simulink model "G_actuatordynamics"  (R2017a)
settings: Solver=FixedStepAuto  StartTime=0.0  StopTime=10  FixedStep=sim_time  RelTol=1e-3  EnableMultiTasking=on
values from neighbouring files (symbols this model uses):
  B = [1 0.5 -0.5 -1 0 0.5 ; 0 0 0 0 2 0 ; -0.05 -0.02 0.02 0.05 0 2 ; -1 -1 -1 -1 -2 0]    [A_runSimulation.m]    (also in C_runSimulation.m; D_runSimulation.m; E_runSimulation.m; F_runSimulation.m)
  gain_four = rand()*2    [A_runSimulation.m]    (also in C_runSimulation.m = 0; D_runSimulation.m; E_runSimulation.m = 0; F_runSimulation.m = 0)
  gain_one = rand()*2    [A_runSimulation.m]    (also in C_runSimulation.m = 0; D_runSimulation.m; E_runSimulation.m = 0; F_runSimulation.m = 0)
  gain_three = rand()*2    [A_runSimulation.m]    (also in C_runSimulation.m = 0; D_runSimulation.m; E_runSimulation.m = 0; F_runSimulation.m = 0)
  gain_two = rand()*2    [A_runSimulation.m]    (also in C_runSimulation.m = 0; D_runSimulation.m; E_runSimulation.m = 0; F_runSimulation.m = 0)
  seed_four = k + 30    [A_runSimulation.m]    (also in C_runSimulation.m; D_runSimulation.m; E_runSimulation.m; F_runSimulation.m)
  seed_one = k    [A_runSimulation.m]    (also in C_runSimulation.m; D_runSimulation.m; E_runSimulation.m; F_runSimulation.m)
  seed_three = k + 20    [A_runSimulation.m]    (also in C_runSimulation.m; D_runSimulation.m; E_runSimulation.m; F_runSimulation.m)
  seed_two = k + 10    [A_runSimulation.m]    (also in C_runSimulation.m; D_runSimulation.m; E_runSimulation.m; F_runSimulation.m)
  signal_gain = j    [A_runSimulation.m]    (also in C_runSimulation.m; D_runSimulation.m; E_runSimulation.m = 0.3; F_runSimulation.m)
  sim_time = 1    [E_runSimulation.m]    (also in F_runSimulation.m = 0.1; F_runSimulation2.m = 0.1; G_runSimulation.m = 0.001)
  u_lim = [[-0.5 -0.5 -0.5 -0.5 -0.5 -0.5]' [0.5 0.5 0.5 0.5 0.5 0.5]']    [A_runSimulation.m]    (also in C_runSimulation.m; D_runSimulation.m; E_runSimulation.m; F_runSimulation.m)
  udot_lim = [[2 2 2 2 2 2]']    [A_runSimulation.m]    (also in C_runSimulation.m; D_runSimulation.m; E_runSimulation.m; F_runSimulation.m)
  W1 = eye(6)    [G_runSimulation.m]
  W2 = eye(6)    [G_runSimulation.m]
libraries: dspsrcs4 x8
(part 1 of 2)
settings Model: Creator=markvoskuijl  LastModifiedBy=Luca
settings DataIOCC: LimitDataPoints=on  SaveFormat=Array
settings OptimizationCC: ExpressionDepthLimit=2147483647  LifeSpan=inf
settings DebuggingCC: UnderspecifiedInitializationDetection=Classic  MergeDetectMultiDrivingBlocksExec=none  SolverPrmCheckMsg=warning  FcnCallInpInsideContextMsg=warning  StateNameClashWarn=warning  SFUnexpectedBacktrackingDiag=warning  SFNoUnconditionalDefaultTransitionDiag=warning  SFExecutionAtInitializationDiag=none
settings HardwareCC: ProdBitPerPointer=32  ProdBitPerSizeT=32  ProdBitPerPtrDiffT=32  ProdLargestAtomicFloat=None  ProdIntDivRoundTo=Undefined  ProdEndianess=Unspecified  ProdWordSize=32  ProdHWDeviceType=32-bit Generic
settings ModelReferenceCC: PropagateSignalLabelsOutOfModel=off
settings GRTTargetCC: TargetLangStandard=C89/C90 (ANSI)  GeneratePreprocessorConditionals=Disable all  CombineOutputUpdateFcns=off  GRTInterface=on
settings ConfigComp: CovMetricSettings=dw  CovHtmlReporting=on  CovSaveCumulativeToWorkspaceVar=on  CovSaveSingleToWorkspaceVar=on  CovExternalEMLEnable=off

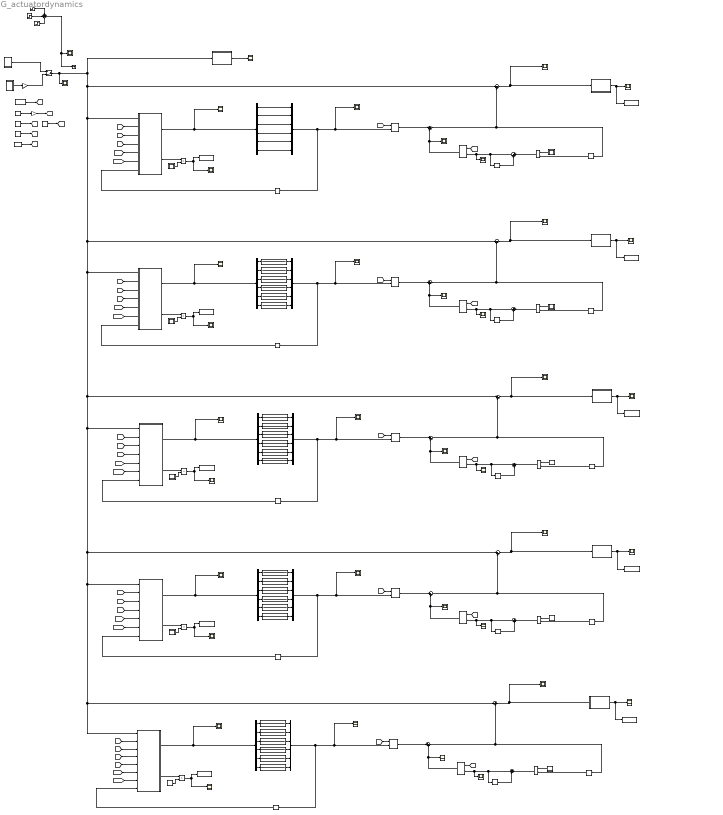
== system G_actuatordynamics ==
  note: all fast w=100
  note: all slow w=10
  note: 2,3,6 slow w=1
  note: 2,3,6 slow w=1
      | compensated
      | harkegard
  A1 : Constant  Value=[-1 0 0.1 0 ; 0 -1 0 -0.1 ; 0 0 -1 0 ; 0 -0.1 0 -1] *0.1
  Constant1 : Constant  Value=W2
  Constant10 : Constant  Value=u_lim
  Constant14 : Constant  Value=B
  Constant4 : Constant  Value=W1
  Demux{,1..4} (5 alike) : Demux  Outputs=6
  FRAMEWISE CONTROL ALLOCATION simple pseudoinverse : Subsystem
  FRAMEWISE CONTROL ALLOCATION simple pseudoinverse1 : Subsystem
  FRAMEWISE CONTROL ALLOCATION simple pseudoinverse2 : Subsystem
  FRAMEWISE CONTROL ALLOCATION simple pseudoinverse3 : Subsystem
  FRAMEWISE CONTROL ALLOCATION simple pseudoinverse4 : Subsystem
  Gain : Gain  Gain=0.01
  Gain4 : Gain  Gain=signal_gain
  Manual Switch : ManualSwitch  CurrentSetting=0
  Matrix Multiply{1..10} (10 alike) : Product  Multiplication=Matrix(*)
  Memory{,1,5,9,14} (5 alike) : Memory  X0=[0 0 0 0 0 0]'
  Memory{2..4,6..8,10..13} (10 alike) : Memory  X0=[0 0 0 0]
  Mux{,1..4} (5 alike) : Mux  Inputs=6
  Product{1..10} (10 alike) : Product
  Scope{,1..37} (38 alike) : Scope
  Step : Step  Time=50  Before=1  After=0  SampleTime=0
  Step1 : Step  Time=100  SampleTime=0
  Step2 : Step  Time=150  SampleTime=0
  Sum : Sum  Inputs=++-
  Sum{1..2,7,10,13} (5 alike) : Sum  Inputs=|-+
  Sum{3..6,8..9,11..12,14..15} (10 alike) : Sum  Inputs=|++
  Terminator : Terminator
  To Workspace1 : ToWorkspace  VariableName=error_base  SampleTime=-1
      settings: Save2DSignal=2-D array (concatenate along first dimension)
  To Workspace10 : ToWorkspace  VariableName=saturatedtime_compensated4  SampleTime=-1
      settings: Save2DSignal=2-D array (concatenate along first dimension)
  To Workspace2 : ToWorkspace  VariableName=error_fast  SampleTime=-1
      settings: Save2DSignal=2-D array (concatenate along first dimension)
  To Workspace3 : ToWorkspace  VariableName=saturatedtime_compensated  SampleTime=-1
      settings: Save2DSignal=2-D array (concatenate along first dimension)
  To Workspace4 : ToWorkspace  VariableName=saturatedtime_compensated1  SampleTime=-1
      settings: Save2DSignal=2-D array (concatenate along first dimension)
  To Workspace5 : ToWorkspace  VariableName=error_slow  SampleTime=-1
      settings: Save2DSignal=2-D array (concatenate along first dimension)
  To Workspace6 : ToWorkspace  VariableName=saturatedtime_compensated2  SampleTime=-1
      settings: Save2DSignal=2-D array (concatenate along first dimension)
  To Workspace7 : ToWorkspace  VariableName=error_half  SampleTime=-1
      settings: Save2DSignal=2-D array (concatenate along first dimension)
  To Workspace8 : ToWorkspace  VariableName=saturatedtime_compensated3  SampleTime=-1
      settings: Save2DSignal=2-D array (concatenate along first dimension)
  To Workspace9 : ToWorkspace  VariableName=error_half_compensated  SampleTime=-1
      settings: Save2DSignal=2-D array (concatenate along first dimension)
  Transfer Fcn Fast{1..5,12..15,19..21} (12 alike) : TransferFcn  Numerator=[(2*pi*10)^2]  Denominator="[1  2*0.9*(2*pi*10)   (2*pi*10)^2]"
  Transfer Fcn Fast{6..11,16..18,22..24} (12 alike) : TransferFcn  Numerator=[(2*pi*100)^2]  Denominator="[1  2*0.9*(2*pi*100)   (2*pi*100)^2]"
  dt1 : Subsystem
  dt10 : Subsystem
  dt2 : Subsystem
  dt3 : Subsystem
  dt4 : Subsystem
  dt5 : Subsystem
  dt6 : Subsystem
  dt7 : Subsystem
  dt8 : Subsystem
  dt9 : Subsystem
  error1 : MATLAB Function  TreatAsAtomicUnit=on
  error2 : MATLAB Function  TreatAsAtomicUnit=on
  error3 : MATLAB Function  TreatAsAtomicUnit=on
  error4 : MATLAB Function  TreatAsAtomicUnit=on
  error5 : MATLAB Function  TreatAsAtomicUnit=on
  error6 : MATLAB Function  TreatAsAtomicUnit=on
  pink noise : Subsystem
  udot lim rad/sec3 : Constant  Value=udot_lim
  white noise : Subsystem
  wires:
  Constant10/1 -> [u_lim]
  Constant4/1 -> [W1]
  pink noise/1(Out1) -> Gain4/1
  white noise/1(Out1) -> Manual Switch/1
  udot lim rad/sec3/1 -> [udot_lim]
  Constant14/1 -> [B]
  Gain4/1 -> Manual Switch/2
  A1/1 -> Gain/1
  Sum5/1 -> Memory4/1, Sum2/2  "acceleration(t)"
  Memory4/1 -> Product1/2  "ccelerations(t-1)"
  [A] -> Matrix Multiply3/1
  [B] -> FRAMEWISE CONTROL ALLOCATION simple pseudoinverse/2(B linearized)
  Matrix Multiply3/1 -> Scope10/1, Sum5/2  "accelerations due to state(t)"
  Sum2/1 -> Scope5/1, error1/1(e)
  Product4/1 -> Scope11/1, To Workspace4/1
  FRAMEWISE CONTROL ALLOCATION simple pseudoinverse/2(saturated(t)) -> Product4/1
  dt4/1(dt) -> Product4/2
  [B] -> Matrix Multiply1/1
  Memory6/1 -> Sum6/2  "state(t-1)"
  dt3/1(dt) -> Product1/1
  [udot_lim] -> FRAMEWISE CONTROL ALLOCATION simple pseudoinverse/6(rate limits)
  [A] -> FRAMEWISE CONTROL ALLOCATION simple pseudoinverse/3(A linearized)
  [u_lim] -> FRAMEWISE CONTROL ALLOCATION simple pseudoinverse/5(deflection limits)
  Matrix Multiply1/1 -> Sum5/1  "accelerations due to deflection(t)"
  error1/1(error) -> Scope12/1, To Workspace1/1
  [W1] -> FRAMEWISE CONTROL ALLOCATION simple pseudoinverse/4(weights matrix)
  Sum6/1 -> Memory6/1, Scope13/1, Matrix Multiply3/2  "state (t)"
  Product1/1 -> Sum6/1  "state variation in dt"
  FRAMEWISE CONTROL ALLOCATION simple pseudoinverse/1(deflections(t)) -> Scope/1, Demux/1  "delta(t)"
  Step/1 -> Sum/1
  Step1/1 -> Sum/2
  Sum/1 -> Terminator/1, Scope14/1
  Step2/1 -> Sum/3
  Gain/1 -> [A]
  Mux/1 -> Scope1/1, Matrix Multiply1/2, Memory/1
  error2/1(error) -> Scope2/1
  Constant1/1 -> [W2]
  Memory/1 -> FRAMEWISE CONTROL ALLOCATION simple pseudoinverse/7(deflections(t-1))
  [udot_lim] -> FRAMEWISE CONTROL ALLOCATION simple pseudoinverse1/6(rate limits)
  Transfer Fcn Fast8/1 -> Mux1/3
  Sum4/1 -> Memory3/1, Scope16/1, Matrix Multiply4/2  "state (t)"
  Transfer Fcn Fast11/1 -> Mux1/6
  Product3/1 -> Scope9/1, To Workspace3/1
  dt1/1(dt) -> Product2/1
  Demux1/5 -> Transfer Fcn Fast10/1
  Transfer Fcn Fast9/1 -> Mux1/4
  Transfer Fcn Fast7/1 -> Mux1/2
  Product2/1 -> Sum4/1  "state variation in dt"
  Demux1/2 -> Transfer Fcn Fast7/1
  [A] -> FRAMEWISE CONTROL ALLOCATION simple pseudoinverse1/3(A linearized)
  dt2/1(dt) -> Product3/2
  Demux1/4 -> Transfer Fcn Fast9/1
  [u_lim] -> FRAMEWISE CONTROL ALLOCATION simple pseudoinverse1/5(deflection limits)
  Memory3/1 -> Sum4/2  "state(t-1)"
  [B] -> FRAMEWISE CONTROL ALLOCATION simple pseudoinverse1/2(B linearized)
  FRAMEWISE CONTROL ALLOCATION simple pseudoinverse1/1(deflections(t)) -> Scope4/1, Demux1/1  "delta(t)"
  FRAMEWISE CONTROL ALLOCATION simple pseudoinverse1/2(saturated(t)) -> Product3/1
  Sum1/1 -> Scope19/1, error3/1(e)
  Sum3/1 -> Memory2/1, Sum1/2  "acceleration(t)"
  [B] -> Matrix Multiply2/1
  [A] -> Matrix Multiply4/1
  Demux1/1 -> Transfer Fcn Fast6/1
  Transfer Fcn Fast6/1 -> Mux1/1
  [W1] -> FRAMEWISE CONTROL ALLOCATION simple pseudoinverse1/4(weights matrix)
  Matrix Multiply2/1 -> Sum3/1  "accelerations due to deflection(t)"
  Matrix Multiply4/1 -> Scope8/1, Sum3/2  "accelerations due to state(t)"
  Memory1/1 -> FRAMEWISE CONTROL ALLOCATION simple pseudoinverse1/7(deflections(t-1))
  error3/1(error) -> To Workspace2/1, Scope15/1
  Memory2/1 -> Product2/2  "ccelerations(t-1)"
  Demux1/6 -> Transfer Fcn Fast11/1
  Demux1/3 -> Transfer Fcn Fast8/1
  Mux1/1 -> Scope6/1, Matrix Multiply2/2, Memory1/1
  Transfer Fcn Fast10/1 -> Mux1/5
  Demux/1 -> Mux/1
  Demux/2 -> Mux/2
  Demux/3 -> Mux/3
  Demux/4 -> Mux/4
  Demux/5 -> Mux/5
  Demux/6 -> Mux/6
  Matrix Multiply6/1 -> Scope26/1, Sum8/2  "accelerations due to state(t)"
  Memory5/1 -> FRAMEWISE CONTROL ALLOCATION simple pseudoinverse2/7(deflections(t-1))
  error4/1(error) -> To Workspace5/1, Scope18/1
  FRAMEWISE CONTROL ALLOCATION simple pseudoinverse2/2(saturated(t)) -> Product6/1
  [W1] -> FRAMEWISE CONTROL ALLOCATION simple pseudoinverse2/4(weights matrix)
  Transfer Fcn Fast3/1 -> Mux2/1
  Sum8/1 -> Memory7/1, Sum7/2  "acceleration(t)"
  Memory7/1 -> Product5/2  "ccelerations(t-1)"
  Mux2/1 -> Scope25/1, Matrix Multiply5/2, Memory5/1
  Sum7/1 -> Scope22/1, error4/1(e)
  [B] -> Matrix Multiply5/1
  Product6/1 -> Scope27/1, To Workspace6/1
  Product5/1 -> Sum9/1  "state variation in dt"
  [B] -> FRAMEWISE CONTROL ALLOCATION simple pseudoinverse2/2(B linearized)
  Sum9/1 -> Memory8/1, Scope21/1, Matrix Multiply6/2  "state (t)"
  dt5/1(dt) -> Product5/1
  [A] -> Matrix Multiply6/1
  FRAMEWISE CONTROL ALLOCATION simple pseudoinverse2/1(deflections(t)) -> Scope24/1, Demux2/1  "delta(t)"
  dt6/1(dt) -> Product6/2
  [A] -> FRAMEWISE CONTROL ALLOCATION simple pseudoinverse2/3(A linearized)
  Memory8/1 -> Sum9/2  "state(t-1)"
  [udot_lim] -> FRAMEWISE CONTROL ALLOCATION simple pseudoinverse2/6(rate limits)
  Matrix Multiply5/1 -> Sum8/1  "accelerations due to deflection(t)"
  [u_lim] -> FRAMEWISE CONTROL ALLOCATION simple pseudoinverse2/5(deflection limits)
  Demux2/1 -> Transfer Fcn Fast3/1
  [A] -> FRAMEWISE CONTROL ALLOCATION simple pseudoinverse3/3(A linearized)
  FRAMEWISE CONTROL ALLOCATION simple pseudoinverse3/1(deflections(t)) -> Scope20/1, Demux3/1  "delta(t)"
  [A] -> Matrix Multiply8/1
  dt7/1(dt) -> Product7/1
  [udot_lim] -> FRAMEWISE CONTROL ALLOCATION simple pseudoinverse3/6(rate limits)
  [B] -> FRAMEWISE CONTROL ALLOCATION simple pseudoinverse3/2(B linearized)
  Product7/1 -> Sum12/1  "state variation in dt"
  Product8/1 -> Scope29/1, To Workspace8/1
  [B] -> Matrix Multiply7/1
  Sum10/1 -> Scope30/1, error5/1(e)
  Memory11/1 -> Sum12/2  "state(t-1)"
  Mux3/1 -> Scope23/1, Matrix Multiply7/2, Memory9/1
  Transfer Fcn Fast16/1 -> Mux3/1
  Memory10/1 -> Product7/2  "ccelerations(t-1)"
  [W1] -> FRAMEWISE CONTROL ALLOCATION simple pseudoinverse3/4(weights matrix)
  dt8/1(dt) -> Product8/2
  Memory9/1 -> FRAMEWISE CONTROL ALLOCATION simple pseudoinverse3/7(deflections(t-1))
  error5/1(error) -> To Workspace7/1, Scope7/1
  Matrix Multiply8/1 -> Scope28/1, Sum11/2  "accelerations due to state(t)"
  Demux3/1 -> Transfer Fcn Fast16/1
  Demux3/3 -> Transfer Fcn Fast15/1
  [u_lim] -> FRAMEWISE CONTROL ALLOCATION simple pseudoinverse3/5(deflection limits)
  Matrix Multiply7/1 -> Sum11/1  "accelerations due to deflection(t)"
  Transfer Fcn Fast14/1 -> Mux3/6
  Transfer Fcn Fast15/1 -> Mux3/3
  Demux3/6 -> Transfer Fcn Fast14/1
  Transfer Fcn Fast17/1 -> Mux3/4
  Demux3/4 -> Transfer Fcn Fast17/1
  Transfer Fcn Fast18/1 -> Mux3/5
  Demux3/5 -> Transfer Fcn Fast18/1
  FRAMEWISE CONTROL ALLOCATION simple pseudoinverse3/2(saturated(t)) -> Product8/1
  Sum12/1 -> Memory11/1, Scope17/1, Matrix Multiply8/2  "state (t)"
  Demux3/2 -> Transfer Fcn Fast13/1
  Sum11/1 -> Memory10/1, Sum10/2  "acceleration(t)"
  Transfer Fcn Fast13/1 -> Mux3/2
  error6/1(error) -> To Workspace9/1, Scope36/1
  Memory14/1 -> FRAMEWISE CONTROL ALLOCATION simple pseudoinverse4/8(deflections(t-1))
  Sum14/1 -> Memory12/1, Sum13/2  "acceleration(t)"
  Sum15/1 -> Memory13/1, Scope31/1, Matrix Multiply10/2  "state (t)"
  [u_lim] -> FRAMEWISE CONTROL ALLOCATION simple pseudoinverse4/6(deflection limits)
  Manual Switch/1 -> error2/1(e), Sum7/1, Sum10/1, FRAMEWISE CONTROL ALLOCATION simple pseudoinverse4/1(virtual control), Sum13/1, FRAMEWISE CONTROL ALLOCATION simple pseudoinverse3/1(virtual control), FRAMEWISE CONTROL ALLOCATION simple pseudoinverse2/1(virtual control), FRAMEWISE CONTROL ALLOCATION simple pseudoinverse1/1(virtual control), Sum1/1, FRAMEWISE CONTROL ALLOCATION simple pseudoinverse/1(virtual control), Sum2/1, Scope3/1
  Product9/1 -> Sum15/1  "state variation in dt"
  [B] -> FRAMEWISE CONTROL ALLOCATION simple pseudoinverse4/2(B linearized)
  dt9/1(dt) -> Product9/1
  [udot_lim] -> FRAMEWISE CONTROL ALLOCATION simple pseudoinverse4/7(rate limits)
  FRAMEWISE CONTROL ALLOCATION simple pseudoinverse4/1(deflections(t)) -> Scope32/1, Demux4/1  "delta(t)"
  [A] -> Matrix Multiply10/1
  Matrix Multiply10/1 -> Scope34/1, Sum14/2  "accelerations due to state(t)"
  [W1] -> FRAMEWISE CONTROL ALLOCATION simple pseudoinverse4/4(weights deflection)
  Matrix Multiply9/1 -> Sum14/1  "accelerations due to deflection(t)"
  Memory12/1 -> Product9/2  "ccelerations(t-1)"
  Mux4/1 -> Scope33/1, Matrix Multiply9/2, Memory14/1
  dt10/1(dt) -> Product10/2
  Memory13/1 -> Sum15/2  "state(t-1)"
  Product10/1 -> Scope35/1, To Workspace10/1
  [B] -> Matrix Multiply9/1
  [A] -> FRAMEWISE CONTROL ALLOCATION simple pseudoinverse4/3(A linearized)
  Sum13/1 -> Scope37/1, error6/1(e)
  FRAMEWISE CONTROL ALLOCATION simple pseudoinverse4/2(saturated(t)) -> Product10/1
  [W2] -> FRAMEWISE CONTROL ALLOCATION simple pseudoinverse4/5(weights rate)
  Demux2/2 -> Transfer Fcn Fast1/1
  Transfer Fcn Fast1/1 -> Mux2/2
  Demux2/3 -> Transfer Fcn Fast4/1
  Transfer Fcn Fast4/1 -> Mux2/3
  Transfer Fcn Fast2/1 -> Mux2/4
  Demux2/4 -> Transfer Fcn Fast2/1
  Demux2/5 -> Transfer Fcn Fast12/1
  Transfer Fcn Fast12/1 -> Mux2/5
  Transfer Fcn Fast5/1 -> Mux2/6
  Demux2/6 -> Transfer Fcn Fast5/1
  Transfer Fcn Fast24/1 -> Mux4/5
  Demux4/1 -> Transfer Fcn Fast22/1
  Transfer Fcn Fast21/1 -> Mux4/3
  Demux4/4 -> Transfer Fcn Fast23/1
  Transfer Fcn Fast23/1 -> Mux4/4
  Transfer Fcn Fast20/1 -> Mux4/6
  Demux4/6 -> Transfer Fcn Fast20/1
  Demux4/5 -> Transfer Fcn Fast24/1
  Demux4/3 -> Transfer Fcn Fast21/1
  Transfer Fcn Fast22/1 -> Mux4/1
  Demux4/2 -> Transfer Fcn Fast19/1
  Transfer Fcn Fast19/1 -> Mux4/2

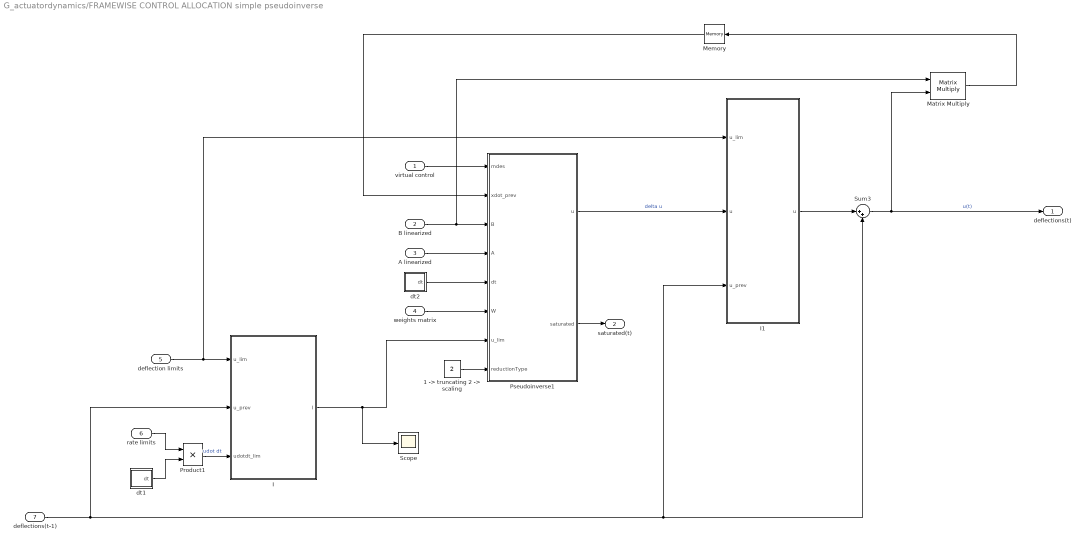
== system G_actuatordynamics/FRAMEWISE CONTROL ALLOCATION simple pseudoinverse ==
  virtual control : Inport
  B linearized : Inport  Port=2
  A linearized : Inport  Port=3
  weights matrix : Inport  Port=4
  deflection limits : Inport  Port=5
  rate limits : Inport  Port=6
  deflections(t-1) : Inport  Port=7
  "1 -> truncating 2 -> scaling" : Constant  Value=2
  I : MATLAB Function  TreatAsAtomicUnit=on
  I1 : MATLAB Function  TreatAsAtomicUnit=on
  Matrix Multiply : Product  Multiplication=Matrix(*)
  Memory : Memory  X0=[0 0 0 0]'
  Product1 : Product
  Pseudoinverse1 : MATLAB Function  TreatAsAtomicUnit=on
  Scope : Scope
  Sum3 : Sum  Inputs=|++
  dt1 : Subsystem
  dt2 : Subsystem
  deflections(t) : Outport
  saturated(t) : Outport  Port=2
  wires:
  I/1(I) -> Scope/1, Pseudoinverse1/7(u_lim)
  Product1/1 -> I/3(udotdt_lim)  "udot dt"
  rate limits/1 -> Product1/1
  Sum3/1 -> Matrix Multiply/2, deflections(t)/1  "u(t)"
  B linearized/1 -> Matrix Multiply/1, Pseudoinverse1/3(B)
  deflection limits/1 -> I1/1(u_lim), I/1(u_lim)
  weights matrix/1 -> Pseudoinverse1/6(W)
  "1 -> truncating 2 -> scaling"/1 -> Pseudoinverse1/8(reductionType)
  virtual control/1 -> Pseudoinverse1/1(mdes)
  Matrix Multiply/1 -> Memory/1
  dt2/1(dt) -> Pseudoinverse1/5(dt)
  A linearized/1 -> Pseudoinverse1/4(A)
  dt1/1(dt) -> Product1/2
  Pseudoinverse1/2(saturated) -> saturated(t)/1
  deflections(t-1)/1 -> I1/3(u_prev), Sum3/2, I/2(u_prev)
  I1/1(u) -> Sum3/1
  Pseudoinverse1/1(u) -> I1/2("u ")  "delta u"
  Memory/1 -> Pseudoinverse1/2(xdot_prev)

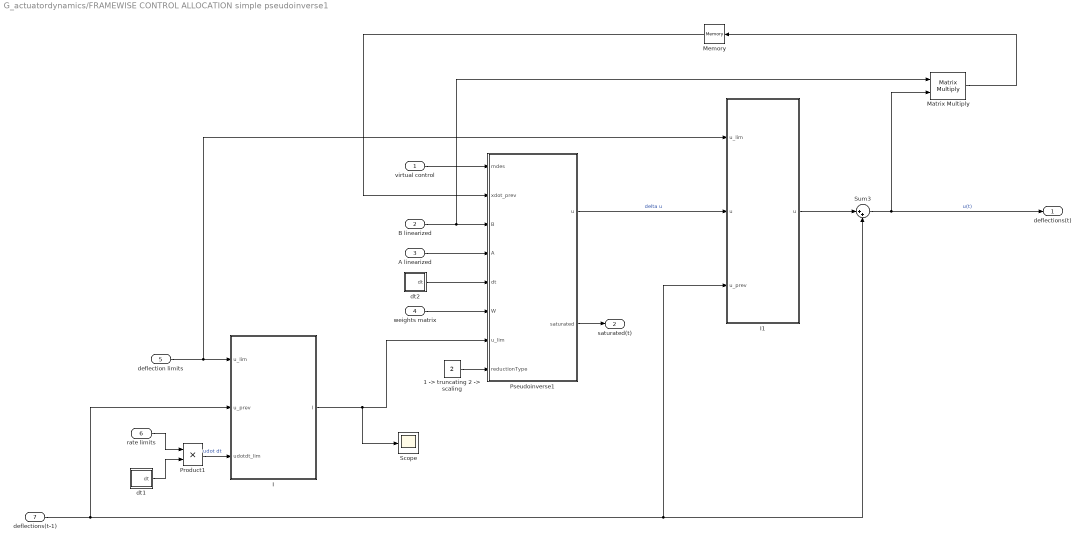
== system G_actuatordynamics/FRAMEWISE CONTROL ALLOCATION simple pseudoinverse1 ==
  virtual control : Inport
  B linearized : Inport  Port=2
  A linearized : Inport  Port=3
  weights matrix : Inport  Port=4
  deflection limits : Inport  Port=5
  rate limits : Inport  Port=6
  deflections(t-1) : Inport  Port=7
  "1 -> truncating 2 -> scaling" : Constant  Value=2
  I : MATLAB Function  TreatAsAtomicUnit=on
  I1 : MATLAB Function  TreatAsAtomicUnit=on
  Matrix Multiply : Product  Multiplication=Matrix(*)
  Memory : Memory  X0=[0 0 0 0]'
  Product1 : Product
  Pseudoinverse1 : MATLAB Function  TreatAsAtomicUnit=on
  Scope : Scope
  Sum3 : Sum  Inputs=|++
  dt1 : Subsystem
  dt2 : Subsystem
  deflections(t) : Outport
  saturated(t) : Outport  Port=2
  wires:
  I/1(I) -> Scope/1, Pseudoinverse1/7(u_lim)
  Product1/1 -> I/3(udotdt_lim)  "udot dt"
  rate limits/1 -> Product1/1
  Sum3/1 -> Matrix Multiply/2, deflections(t)/1  "u(t)"
  B linearized/1 -> Matrix Multiply/1, Pseudoinverse1/3(B)
  deflection limits/1 -> I1/1(u_lim), I/1(u_lim)
  weights matrix/1 -> Pseudoinverse1/6(W)
  "1 -> truncating 2 -> scaling"/1 -> Pseudoinverse1/8(reductionType)
  virtual control/1 -> Pseudoinverse1/1(mdes)
  Matrix Multiply/1 -> Memory/1
  dt2/1(dt) -> Pseudoinverse1/5(dt)
  A linearized/1 -> Pseudoinverse1/4(A)
  dt1/1(dt) -> Product1/2
  Pseudoinverse1/2(saturated) -> saturated(t)/1
  deflections(t-1)/1 -> I1/3(u_prev), Sum3/2, I/2(u_prev)
  I1/1(u) -> Sum3/1
  Pseudoinverse1/1(u) -> I1/2("u ")  "delta u"
  Memory/1 -> Pseudoinverse1/2(xdot_prev)

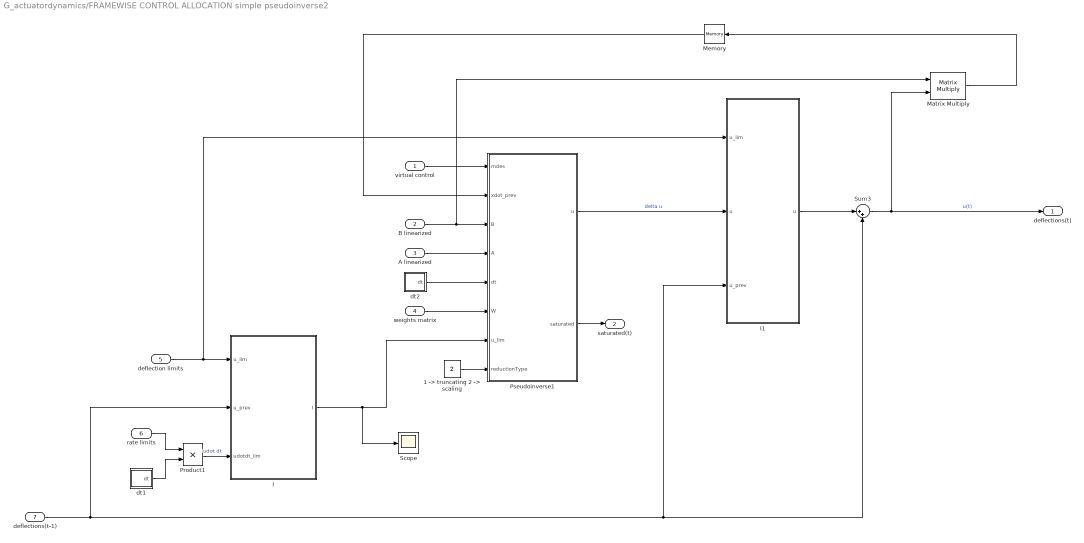
== system G_actuatordynamics/FRAMEWISE CONTROL ALLOCATION simple pseudoinverse2 ==
  virtual control : Inport
  B linearized : Inport  Port=2
  A linearized : Inport  Port=3
  weights matrix : Inport  Port=4
  deflection limits : Inport  Port=5
  rate limits : Inport  Port=6
  deflections(t-1) : Inport  Port=7
  "1 -> truncating 2 -> scaling" : Constant  Value=2
  I : MATLAB Function  TreatAsAtomicUnit=on
  I1 : MATLAB Function  TreatAsAtomicUnit=on
  Matrix Multiply : Product  Multiplication=Matrix(*)
  Memory : Memory  X0=[0 0 0 0]'
  Product1 : Product
  Pseudoinverse1 : MATLAB Function  TreatAsAtomicUnit=on
  Scope : Scope
  Sum3 : Sum  Inputs=|++
  dt1 : Subsystem
  dt2 : Subsystem
  deflections(t) : Outport
  saturated(t) : Outport  Port=2
  wires:
  I/1(I) -> Scope/1, Pseudoinverse1/7(u_lim)
  Product1/1 -> I/3(udotdt_lim)  "udot dt"
  rate limits/1 -> Product1/1
  Sum3/1 -> Matrix Multiply/2, deflections(t)/1  "u(t)"
  B linearized/1 -> Matrix Multiply/1, Pseudoinverse1/3(B)
  deflection limits/1 -> I1/1(u_lim), I/1(u_lim)
  weights matrix/1 -> Pseudoinverse1/6(W)
  "1 -> truncating 2 -> scaling"/1 -> Pseudoinverse1/8(reductionType)
  virtual control/1 -> Pseudoinverse1/1(mdes)
  Matrix Multiply/1 -> Memory/1
  dt2/1(dt) -> Pseudoinverse1/5(dt)
  A linearized/1 -> Pseudoinverse1/4(A)
  dt1/1(dt) -> Product1/2
  Pseudoinverse1/2(saturated) -> saturated(t)/1
  deflections(t-1)/1 -> I1/3(u_prev), Sum3/2, I/2(u_prev)
  I1/1(u) -> Sum3/1
  Pseudoinverse1/1(u) -> I1/2("u ")  "delta u"
  Memory/1 -> Pseudoinverse1/2(xdot_prev)

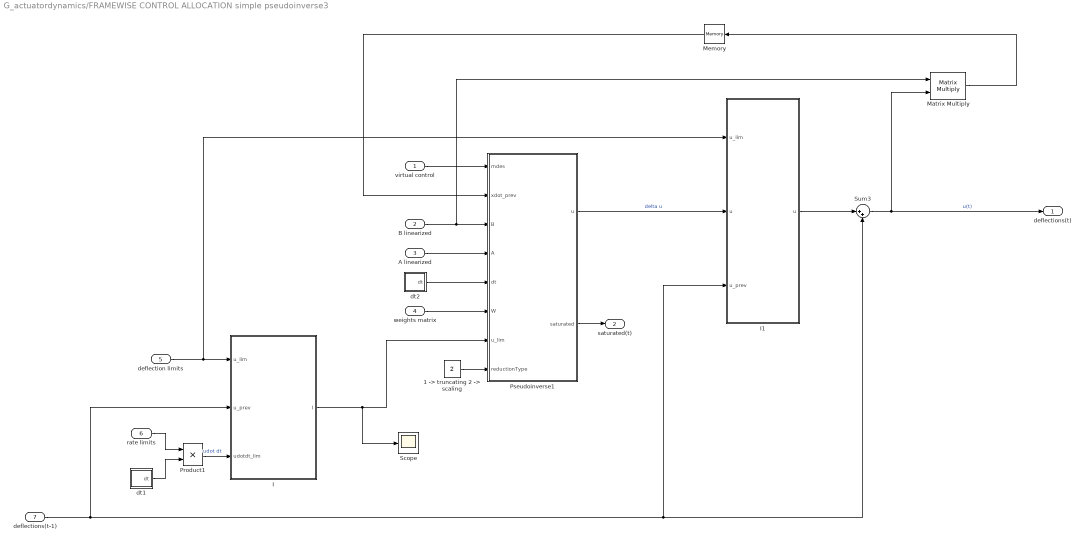
== system G_actuatordynamics/FRAMEWISE CONTROL ALLOCATION simple pseudoinverse3 ==
  virtual control : Inport
  B linearized : Inport  Port=2
  A linearized : Inport  Port=3
  weights matrix : Inport  Port=4
  deflection limits : Inport  Port=5
  rate limits : Inport  Port=6
  deflections(t-1) : Inport  Port=7
  "1 -> truncating 2 -> scaling" : Constant  Value=2
  I : MATLAB Function  TreatAsAtomicUnit=on
  I1 : MATLAB Function  TreatAsAtomicUnit=on
  Matrix Multiply : Product  Multiplication=Matrix(*)
  Memory : Memory  X0=[0 0 0 0]'
  Product1 : Product
  Pseudoinverse1 : MATLAB Function  TreatAsAtomicUnit=on
  Scope : Scope
  Sum3 : Sum  Inputs=|++
  dt1 : Subsystem
  dt2 : Subsystem
  deflections(t) : Outport
  saturated(t) : Outport  Port=2
  wires:
  I/1(I) -> Scope/1, Pseudoinverse1/7(u_lim)
  Product1/1 -> I/3(udotdt_lim)  "udot dt"
  rate limits/1 -> Product1/1
  Sum3/1 -> Matrix Multiply/2, deflections(t)/1  "u(t)"
  B linearized/1 -> Matrix Multiply/1, Pseudoinverse1/3(B)
  deflection limits/1 -> I1/1(u_lim), I/1(u_lim)
  weights matrix/1 -> Pseudoinverse1/6(W)
  "1 -> truncating 2 -> scaling"/1 -> Pseudoinverse1/8(reductionType)
  virtual control/1 -> Pseudoinverse1/1(mdes)
  Matrix Multiply/1 -> Memory/1
  dt2/1(dt) -> Pseudoinverse1/5(dt)
  A linearized/1 -> Pseudoinverse1/4(A)
  dt1/1(dt) -> Product1/2
  Pseudoinverse1/2(saturated) -> saturated(t)/1
  deflections(t-1)/1 -> I1/3(u_prev), Sum3/2, I/2(u_prev)
  I1/1(u) -> Sum3/1
  Pseudoinverse1/1(u) -> I1/2("u ")  "delta u"
  Memory/1 -> Pseudoinverse1/2(xdot_prev)

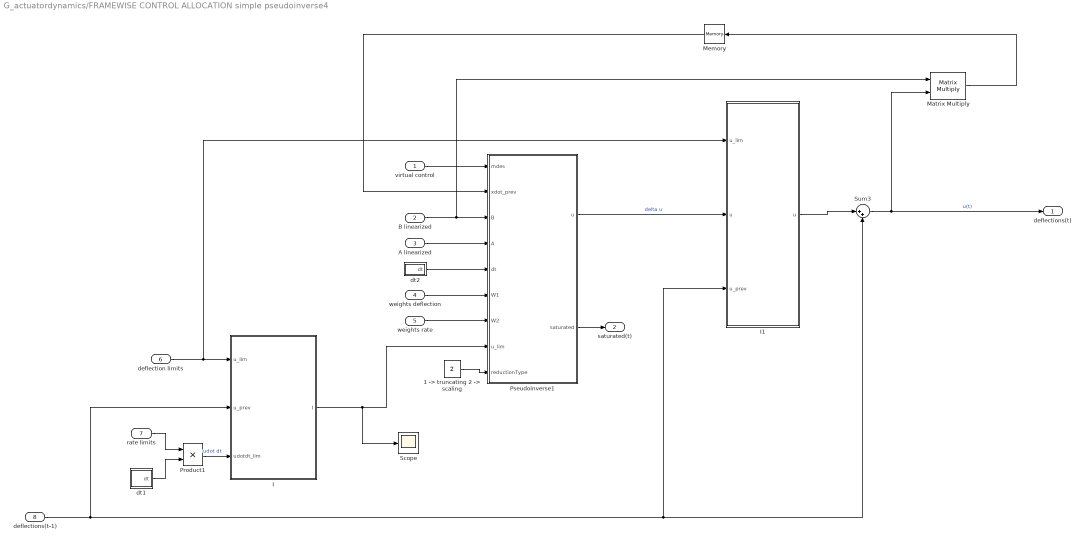
== system G_actuatordynamics/FRAMEWISE CONTROL ALLOCATION simple pseudoinverse4 ==
  virtual control : Inport
  B linearized : Inport  Port=2
  A linearized : Inport  Port=3
  weights deflection : Inport  Port=4
  weights rate : Inport  Port=5
  deflection limits : Inport  Port=6
  rate limits : Inport  Port=7
  deflections(t-1) : Inport  Port=8
  "1 -> truncating 2 -> scaling" : Constant  Value=2
  I : MATLAB Function  TreatAsAtomicUnit=on
  I1 : MATLAB Function  TreatAsAtomicUnit=on
  Matrix Multiply : Product  Multiplication=Matrix(*)
  Memory : Memory  X0=[0 0 0 0]'
  Product1 : Product
  Pseudoinverse1 : MATLAB Function  TreatAsAtomicUnit=on
  Scope : Scope
  Sum3 : Sum  Inputs=|++
  dt1 : Subsystem
  dt2 : Subsystem
  deflections(t) : Outport
  saturated(t) : Outport  Port=2
  wires:
  I/1(I) -> Scope/1, Pseudoinverse1/8(u_lim)
  Product1/1 -> I/3(udotdt_lim)  "udot dt"
  rate limits/1 -> Product1/1
  Sum3/1 -> Matrix Multiply/2, deflections(t)/1  "u(t)"
  B linearized/1 -> Pseudoinverse1/3(B), Matrix Multiply/1
  deflection limits/1 -> I1/1(u_lim), I/1(u_lim)
  weights deflection/1 -> Pseudoinverse1/6(W1)
  "1 -> truncating 2 -> scaling"/1 -> Pseudoinverse1/9(reductionType)
  virtual control/1 -> Pseudoinverse1/1(mdes)
  Matrix Multiply/1 -> Memory/1
  dt2/1(dt) -> Pseudoinverse1/5(dt)
  A linearized/1 -> Pseudoinverse1/4(A)
  dt1/1(dt) -> Product1/2
  Pseudoinverse1/2(saturated) -> saturated(t)/1
  deflections(t-1)/1 -> I1/3(u_prev), Sum3/2, I/2(u_prev)
  I1/1(u) -> Sum3/1
  Pseudoinverse1/1(u) -> I1/2("u ")  "delta u"
  Memory/1 -> Pseudoinverse1/2(xdot_prev)
  weights rate/1 -> Pseudoinverse1/7(W2)

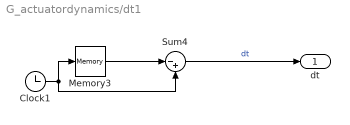
== system G_actuatordynamics/dt1 ==
  Clock1 : Clock
  Memory3 : Memory
  Sum4 : Sum  Inputs=|-+
  dt : Outport
  wires:
  Clock1/1 -> Sum4/2, Memory3/1
  Memory3/1 -> Sum4/1
  Sum4/1 -> dt/1  "dt"

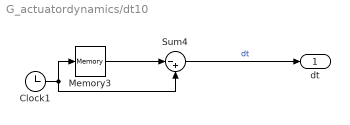
== system G_actuatordynamics/dt10 ==
  Clock1 : Clock
  Memory3 : Memory
  Sum4 : Sum  Inputs=|-+
  dt : Outport
  wires:
  Clock1/1 -> Sum4/2, Memory3/1
  Memory3/1 -> Sum4/1
  Sum4/1 -> dt/1  "dt"

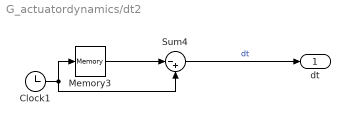
== system G_actuatordynamics/dt2 ==
  Clock1 : Clock
  Memory3 : Memory
  Sum4 : Sum  Inputs=|-+
  dt : Outport
  wires:
  Clock1/1 -> Sum4/2, Memory3/1
  Memory3/1 -> Sum4/1
  Sum4/1 -> dt/1  "dt"

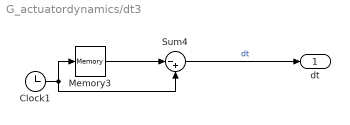
== system G_actuatordynamics/dt3 ==
  Clock1 : Clock
  Memory3 : Memory
  Sum4 : Sum  Inputs=|-+
  dt : Outport
  wires:
  Clock1/1 -> Sum4/2, Memory3/1
  Memory3/1 -> Sum4/1
  Sum4/1 -> dt/1  "dt"

== system G_actuatordynamics/dt4 ==
  Clock1 : Clock
  Memory3 : Memory
  Sum4 : Sum  Inputs=|-+
  dt : Outport
  wires:
  Clock1/1 -> Sum4/2, Memory3/1
  Memory3/1 -> Sum4/1
  Sum4/1 -> dt/1  "dt"

== system G_actuatordynamics/dt5 ==
  Clock1 : Clock
  Memory3 : Memory
  Sum4 : Sum  Inputs=|-+
  dt : Outport
  wires:
  Clock1/1 -> Sum4/2, Memory3/1
  Memory3/1 -> Sum4/1
  Sum4/1 -> dt/1  "dt"

== system G_actuatordynamics/dt6 ==
  Clock1 : Clock
  Memory3 : Memory
  Sum4 : Sum  Inputs=|-+
  dt : Outport
  wires:
  Clock1/1 -> Sum4/2, Memory3/1
  Memory3/1 -> Sum4/1
  Sum4/1 -> dt/1  "dt"

== system G_actuatordynamics/dt7 ==
  Clock1 : Clock
  Memory3 : Memory
  Sum4 : Sum  Inputs=|-+
  dt : Outport
  wires:
  Clock1/1 -> Sum4/2, Memory3/1
  Memory3/1 -> Sum4/1
  Sum4/1 -> dt/1  "dt"

== system G_actuatordynamics/dt8 ==
  Clock1 : Clock
  Memory3 : Memory
  Sum4 : Sum  Inputs=|-+
  dt : Outport
  wires:
  Clock1/1 -> Sum4/2, Memory3/1
  Memory3/1 -> Sum4/1
  Sum4/1 -> dt/1  "dt"

== system G_actuatordynamics/dt9 ==
  Clock1 : Clock
  Memory3 : Memory
  Sum4 : Sum  Inputs=|-+
  dt : Outport
  wires:
  Clock1/1 -> Sum4/2, Memory3/1
  Memory3/1 -> Sum4/1
  Sum4/1 -> dt/1  "dt"

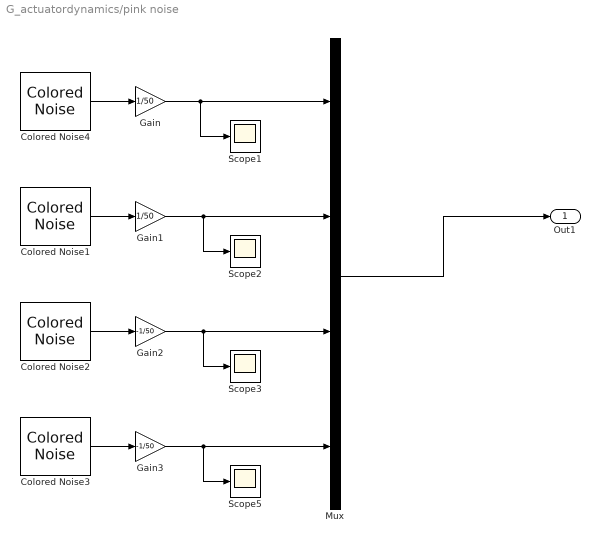
== system G_actuatordynamics/pink noise ==
  Colored Noise1 : dspsrcs4/Colored Noise  Color=custom  InverseFrequencyPower=2  NumChannels=1  OutputDataType=single  SamplesPerFrame=1  SampleTime=sim_time  RandomStream=mt19937ar with seed  Seed=seed_two  SimulateUsing=Interpreted execution
      settings: SourceProductName=DSP System Toolbox  SourceProductBaseCode=DS
  Colored Noise2 : dspsrcs4/Colored Noise  Color=custom  InverseFrequencyPower=2  NumChannels=1  OutputDataType=single  SamplesPerFrame=1  SampleTime=sim_time  RandomStream=mt19937ar with seed  Seed=seed_three  SimulateUsing=Interpreted execution
      settings: SourceProductName=DSP System Toolbox  SourceProductBaseCode=DS
  Colored Noise3 : dspsrcs4/Colored Noise  Color=custom  InverseFrequencyPower=2  NumChannels=1  OutputDataType=single  SamplesPerFrame=1  SampleTime=sim_time  RandomStream=mt19937ar with seed  Seed=seed_four  SimulateUsing=Interpreted execution
      settings: SourceProductName=DSP System Toolbox  SourceProductBaseCode=DS
  Colored Noise4 : dspsrcs4/Colored Noise  Color=custom  InverseFrequencyPower=2  NumChannels=1  OutputDataType=single  SamplesPerFrame=1  SampleTime=sim_time  RandomStream=mt19937ar with seed  Seed=seed_one  SimulateUsing=Interpreted execution
      settings: SourceProductName=DSP System Toolbox  SourceProductBaseCode=DS
  Gain : Gain  Gain=1/50
  Gain1 : Gain  Gain=1/50
  Gain2 : Gain  Gain=-1/50
  Gain3 : Gain  Gain=-1/50
  Mux : Mux
  Scope{1..3,5} (4 alike) : Scope
  Out1 : Outport
  wires:
  Colored Noise4/1 -> Gain/1
  Colored Noise1/1 -> Gain1/1
  Colored Noise2/1 -> Gain2/1
  Gain/1 -> Scope1/1, Mux/1
  Gain1/1 -> Scope2/1, Mux/2
  Gain2/1 -> Scope3/1, Mux/3
  Mux/1 -> Out1/1
  Gain3/1 -> Mux/4, Scope5/1
  Colored Noise3/1 -> Gain3/1

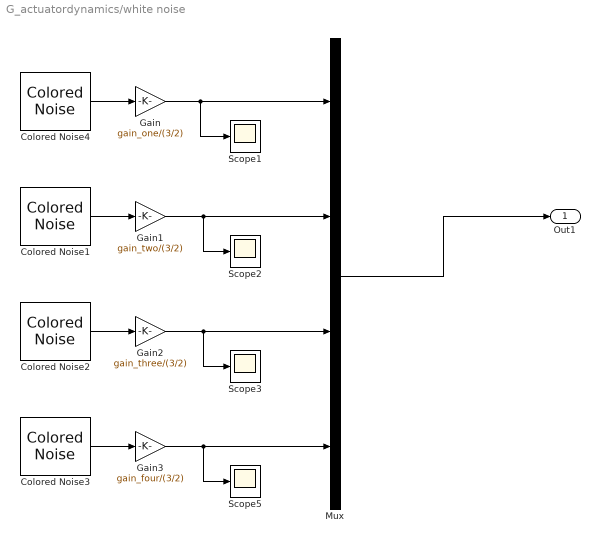
== system G_actuatordynamics/white noise ==
  Colored Noise1 : dspsrcs4/Colored Noise  Color=white  InverseFrequencyPower=2  NumChannels=1  OutputDataType=single  SamplesPerFrame=1  SampleTime=sim_time  RandomStream=mt19937ar with seed  Seed=seed_two  SimulateUsing=Interpreted execution
      settings: SourceProductName=DSP System Toolbox  SourceProductBaseCode=DS
  Colored Noise2 : dspsrcs4/Colored Noise  Color=white  InverseFrequencyPower=2  NumChannels=1  OutputDataType=single  SamplesPerFrame=1  SampleTime=sim_time  RandomStream=mt19937ar with seed  Seed=seed_three  SimulateUsing=Interpreted execution
      settings: SourceProductName=DSP System Toolbox  SourceProductBaseCode=DS
  Colored Noise3 : dspsrcs4/Colored Noise  Color=white  InverseFrequencyPower=2  NumChannels=1  OutputDataType=single  SamplesPerFrame=1  SampleTime=sim_time  RandomStream=mt19937ar with seed  Seed=seed_four  SimulateUsing=Interpreted execution
      settings: SourceProductName=DSP System Toolbox  SourceProductBaseCode=DS
  Colored Noise4 : dspsrcs4/Colored Noise  Color=white  InverseFrequencyPower=2  NumChannels=1  OutputDataType=single  SamplesPerFrame=1  SampleTime=sim_time  RandomStream=mt19937ar with seed  Seed=seed_one  SimulateUsing=Interpreted execution
      settings: SourceProductName=DSP System Toolbox  SourceProductBaseCode=DS
  Gain : Gain  Gain=gain_one/(3/2)
  Gain1 : Gain  Gain=gain_two/(3/2)
  Gain2 : Gain  Gain=gain_three/(3/2)
  Gain3 : Gain  Gain=gain_four/(3/2)
  Mux : Mux
  Scope{1..3,5} (4 alike) : Scope
  Out1 : Outport
  wires:
  Colored Noise4/1 -> Gain/1
  Colored Noise1/1 -> Gain1/1
  Colored Noise2/1 -> Gain2/1
  Gain/1 -> Scope1/1, Mux/1
  Gain1/1 -> Scope2/1, Mux/2
  Gain2/1 -> Scope3/1, Mux/3
  Mux/1 -> Out1/1
  Gain3/1 -> Mux/4, Scope5/1
  Colored Noise3/1 -> Gain3/1

== system G_actuatordynamics/FRAMEWISE CONTROL ALLOCATION simple pseudoinverse/dt1 ==
  Clock1 : Clock
  Memory3 : Memory
  Sum4 : Sum  Inputs=|-+
  dt : Outport
  wires:
  Clock1/1 -> Sum4/2, Memory3/1
  Memory3/1 -> Sum4/1
  Sum4/1 -> dt/1  "dt"

== system G_actuatordynamics/FRAMEWISE CONTROL ALLOCATION simple pseudoinverse/dt2 ==
  Clock1 : Clock
  Memory3 : Memory
  Sum4 : Sum  Inputs=|-+
  dt : Outport
  wires:
  Clock1/1 -> Sum4/2, Memory3/1
  Memory3/1 -> Sum4/1
  Sum4/1 -> dt/1  "dt"

== system G_actuatordynamics/FRAMEWISE CONTROL ALLOCATION simple pseudoinverse1/dt1 ==
  Clock1 : Clock
  Memory3 : Memory
  Sum4 : Sum  Inputs=|-+
  dt : Outport
  wires:
  Clock1/1 -> Sum4/2, Memory3/1
  Memory3/1 -> Sum4/1
  Sum4/1 -> dt/1  "dt"

== system G_actuatordynamics/FRAMEWISE CONTROL ALLOCATION simple pseudoinverse1/dt2 ==
  Clock1 : Clock
  Memory3 : Memory
  Sum4 : Sum  Inputs=|-+
  dt : Outport
  wires:
  Clock1/1 -> Sum4/2, Memory3/1
  Memory3/1 -> Sum4/1
  Sum4/1 -> dt/1  "dt"

== system G_actuatordynamics/FRAMEWISE CONTROL ALLOCATION simple pseudoinverse2/dt1 ==
  Clock1 : Clock
  Memory3 : Memory
  Sum4 : Sum  Inputs=|-+
  dt : Outport
  wires:
  Clock1/1 -> Sum4/2, Memory3/1
  Memory3/1 -> Sum4/1
  Sum4/1 -> dt/1  "dt"

== system G_actuatordynamics/FRAMEWISE CONTROL ALLOCATION simple pseudoinverse2/dt2 ==
  Clock1 : Clock
  Memory3 : Memory
  Sum4 : Sum  Inputs=|-+
  dt : Outport
  wires:
  Clock1/1 -> Sum4/2, Memory3/1
  Memory3/1 -> Sum4/1
  Sum4/1 -> dt/1  "dt"

== system G_actuatordynamics/FRAMEWISE CONTROL ALLOCATION simple pseudoinverse3/dt1 ==
  Clock1 : Clock
  Memory3 : Memory
  Sum4 : Sum  Inputs=|-+
  dt : Outport
  wires:
  Clock1/1 -> Sum4/2, Memory3/1
  Memory3/1 -> Sum4/1
  Sum4/1 -> dt/1  "dt"

== system G_actuatordynamics/FRAMEWISE CONTROL ALLOCATION simple pseudoinverse3/dt2 ==
  Clock1 : Clock
  Memory3 : Memory
  Sum4 : Sum  Inputs=|-+
  dt : Outport
  wires:
  Clock1/1 -> Sum4/2, Memory3/1
  Memory3/1 -> Sum4/1
  Sum4/1 -> dt/1  "dt"

== system G_actuatordynamics/FRAMEWISE CONTROL ALLOCATION simple pseudoinverse4/dt1 ==
  Clock1 : Clock
  Memory3 : Memory
  Sum4 : Sum  Inputs=|-+
  dt : Outport
  wires:
  Clock1/1 -> Sum4/2, Memory3/1
  Memory3/1 -> Sum4/1
  Sum4/1 -> dt/1  "dt"

== system G_actuatordynamics/FRAMEWISE CONTROL ALLOCATION simple pseudoinverse4/dt2 ==
  Clock1 : Clock
  Memory3 : Memory
  Sum4 : Sum  Inputs=|-+
  dt : Outport
  wires:
  Clock1/1 -> Sum4/2, Memory3/1
  Memory3/1 -> Sum4/1
  Sum4/1 -> dt/1  "dt"

== matlab function G_actuatordynamics/error2 ==
  data: e input; error output
function error = error(e)

    error = sum(abs(e));

end

== matlab function G_actuatordynamics/FRAMEWISE CONTROL ALLOCATION simple pseudoinverse1/I ==
  data: u_lim input; u_prev input; udotdt_lim input; I output
function I = computeIntersection(u_lim, u_prev, udotdt_lim)
%check if the matrices are correct
    if not(isequal(size(u_lim,1),size(udotdt_lim,1), size(u_prev,1)))
        error ('input matrix dimensions do not match')
    end

%declare space of intersection
    I = zeros(length(u_lim),2);
    
    I(:,1) = max(-udotdt_lim, u_lim(:,1)-u_prev);
    I(:,2) = min(+udotdt_lim, u_lim(:,2)-u_prev);
    
end

== matlab function G_actuatordynamics/FRAMEWISE CONTROL ALLOCATION simple pseudoinverse1/I1 ==
  data: u_lim input; u input; u output; u_prev input
function u = uCheck(u_lim, u, u_prev)
%check if the matrices are correct
    if not(isequal(size(u_lim,1), size(u,1)))
        error ('input matrix dimensions do not match')
    end

%if computation error occur, correct deflections
    for i = 1:length(u)
        if u(i)+u_prev(i) > u_lim(i,2)
            u(i) = u_lim(i,2)-u_prev(i);
        end
        if u(i)+u_prev(i) < u_lim(i,1)
            u(i) = u_lim(i,1)-u_prev(i);
        end    
    
end

== matlab function G_actuatordynamics/FRAMEWISE CONTROL ALLOCATION simple pseudoinverse/I ==
  data: u_lim input; u_prev input; udotdt_lim input; I output
function I = computeIntersection(u_lim, u_prev, udotdt_lim)
%check if the matrices are correct
    if not(isequal(size(u_lim,1),size(udotdt_lim,1), size(u_prev,1)))
        error ('input matrix dimensions do not match')
    end

%declare space of intersection
    I = zeros(length(u_lim),2);
    
    I(:,1) = max(-udotdt_lim, u_lim(:,1)-u_prev);
    I(:,2) = min(+udotdt_lim, u_lim(:,2)-u_prev);
    
end

== matlab function G_actuatordynamics/FRAMEWISE CONTROL ALLOCATION simple pseudoinverse/I1 ==
  data: u_lim input; u input; u output; u_prev input
function u = uCheck(u_lim, u, u_prev)
%check if the matrices are correct
    if not(isequal(size(u_lim,1), size(u,1)))
        error ('input matrix dimensions do not match')
    end

%if computation error occur, correct deflections
    for i = 1:length(u)
        if u(i)+u_prev(i) > u_lim(i,2)
            u(i) = u_lim(i,2)-u_prev(i);
        end
        if u(i)+u_prev(i) < u_lim(i,1)
            u(i) = u_lim(i,1)-u_prev(i);
        end    
    
end

== matlab function G_actuatordynamics/FRAMEWISE CONTROL ALLOCATION simple pseudoinverse/Pseudoinverse1 ==
  data: mdes input; xdot_prev input; u output; B input; A input; dt input; W input; u_lim input; reductionType input; saturated output
function [u, saturated] = Pseudoinverse(mdes, xdot_prev, B, A, dt, W, u_lim, reductionType)
coder.varsize('u_index', 'Br', 'Wr', 'u_sat');

%check if the matrices are correct
    if not(isequal(size(u_lim,1),size(B,2),size(W,1),size(W,2))...
       && isequal(size(mdes,1),size(B,1),size(A,1),size(A,2),size(xdot_prev,1)))
        error ('input matrix dimensions do not match')
    end
    
%assign to every equation an index    
    u_index = [1:length(u_lim)].';
    I = eye(length(xdot_prev));
    
%compute the remaining moment to compensate
    m = mdes - (I + A*dt)*xdot_prev;
    
%check the type of system and then compute the pseudoinverse 1st step
    order = size(B,2)-size(B,1);

    if order > 0 %over-determined, solution that minimizes the 2norm
        u = inv(W)*B'*inv(B*inv(W)*B')*m;
    elseif order < 0 %under-determined, solution that minimizes the error
        u = inv(B'*B)*B'*m;   
    else %order = 0, sqared thus invertiBrle
        u = inv(B)*m;
    end

%deifne u_sat vector
    u_sat = zeros(length(u),1);
    
    saturated = 0;
%check if the first iteration solution is correct then return    
    if not(any(u <= u_lim(:,1))||any(u >= u_lim(:,2)))  
        return
    end
    
    saturated = 1;
%The software continues only if the solution has to be reduced
%reduce their value
    switch reductionType
        case 1 %truncation
            %takes note of which one are out of their bounds
                u_sat(u < u_lim(:,1)) = 1;
                u_sat(u > u_lim(:,2)) = 1;
                
            %trucate
                u = min(u, u_lim(:,2));
                u = max(u, u_lim(:,1));

        case 2 %scaling solution -> direction preserving
            %reduce
                a = zeros(length(u),1);

                for i = 1:length(u)
                    if u(i)>0
                       a(i) = abs(u(i)/u_lim(i,2));
                    elseif u(i)<0
                       a(i) = abs(u(i)/u_lim(i,1));
                    else
                       a(i) = 0; 
                    end          
                end
                a_max = max(a);
                a_max = max(a_max,1);
                u = u/a_max;
            
            %takes note of which one are out of their bounds
                u_sat(u == u_lim(:,2)) = 1;
                u_sat(u == u_lim(:,1)) = 1;
            
    end
    
return
    
end

== matlab function G_actuatordynamics/error1 ==
  data: e input; error output
function error = error(e)

    error = sum(abs(e));

end

== matlab function G_actuatordynamics/FRAMEWISE CONTROL ALLOCATION simple pseudoinverse1/Pseudoinverse1 ==
  data: mdes input; xdot_prev input; u output; B input; A input; dt input; W input; u_lim input; reductionType input; saturated output
function [u, saturated] = Pseudoinverse(mdes, xdot_prev, B, A, dt, W, u_lim, reductionType)
coder.varsize('u_index', 'Br', 'Wr', 'u_sat');

%check if the matrices are correct
    if not(isequal(size(u_lim,1),size(B,2),size(W,1),size(W,2))...
       && isequal(size(mdes,1),size(B,1),size(A,1),size(A,2),size(xdot_prev,1)))
        error ('input matrix dimensions do not match')
    end
    
%assign to every equation an index    
    u_index = [1:length(u_lim)].';
    I = eye(length(xdot_prev));
    
%compute the remaining moment to compensate
    m = mdes - (I + A*dt)*xdot_prev;
    
%check the type of system and then compute the pseudoinverse 1st step
    order = size(B,2)-size(B,1);

    if order > 0 %over-determined, solution that minimizes the 2norm
        u = inv(W)*B'*inv(B*inv(W)*B')*m;
    elseif order < 0 %under-determined, solution that minimizes the error
        u = inv(B'*B)*B'*m;   
    else %order = 0, sqared thus invertiBrle
        u = inv(B)*m;
    end

%deifne u_sat vector
    u_sat = zeros(length(u),1);
    
    saturated = 0;
%check if the first iteration solution is correct then return    
    if not(any(u <= u_lim(:,1))||any(u >= u_lim(:,2)))  
        return
    end
    
    saturated = 1;
%The software continues only if the solution has to be reduced
%reduce their value
    switch reductionType
        case 1 %truncation
            %takes note of which one are out of their bounds
                u_sat(u < u_lim(:,1)) = 1;
                u_sat(u > u_lim(:,2)) = 1;
                
            %trucate
                u = min(u, u_lim(:,2));
                u = max(u, u_lim(:,1));

        case 2 %scaling solution -> direction preserving
            %reduce
                a = zeros(length(u),1);

                for i = 1:length(u)
                    if u(i)>0
                       a(i) = abs(u(i)/u_lim(i,2));
                    elseif u(i)<0
                       a(i) = abs(u(i)/u_lim(i,1));
                    else
                       a(i) = 0; 
                    end          
                end
                a_max = max(a);
                a_max = max(a_max,1);
                u = u/a_max;
            
            %takes note of which one are out of their bounds
                u_sat(u == u_lim(:,2)) = 1;
                u_sat(u == u_lim(:,1)) = 1;
            
    end
    
return
    
end

== matlab function G_actuatordynamics/error3 ==
  data: e input; error output
function error = error(e)

    error = sum(abs(e));

end

== matlab function G_actuatordynamics/FRAMEWISE CONTROL ALLOCATION simple pseudoinverse2/I ==
  data: u_lim input; u_prev input; udotdt_lim input; I output
function I = computeIntersection(u_lim, u_prev, udotdt_lim)
%check if the matrices are correct
    if not(isequal(size(u_lim,1),size(udotdt_lim,1), size(u_prev,1)))
        error ('input matrix dimensions do not match')
    end

%declare space of intersection
    I = zeros(length(u_lim),2);
    
    I(:,1) = max(-udotdt_lim, u_lim(:,1)-u_prev);
    I(:,2) = min(+udotdt_lim, u_lim(:,2)-u_prev);
    
end

== matlab function G_actuatordynamics/FRAMEWISE CONTROL ALLOCATION simple pseudoinverse2/I1 ==
  data: u_lim input; u input; u output; u_prev input
function u = uCheck(u_lim, u, u_prev)
%check if the matrices are correct
    if not(isequal(size(u_lim,1), size(u,1)))
        error ('input matrix dimensions do not match')
    end

%if computation error occur, correct deflections
    for i = 1:length(u)
        if u(i)+u_prev(i) > u_lim(i,2)
            u(i) = u_lim(i,2)-u_prev(i);
        end
        if u(i)+u_prev(i) < u_lim(i,1)
            u(i) = u_lim(i,1)-u_prev(i);
        end    
    
end

== matlab function G_actuatordynamics/FRAMEWISE CONTROL ALLOCATION simple pseudoinverse2/Pseudoinverse1 ==
  data: mdes input; xdot_prev input; u output; B input; A input; dt input; W input; u_lim input; reductionType input; saturated output
function [u, saturated] = Pseudoinverse(mdes, xdot_prev, B, A, dt, W, u_lim, reductionType)
coder.varsize('u_index', 'Br', 'Wr', 'u_sat');

%check if the matrices are correct
    if not(isequal(size(u_lim,1),size(B,2),size(W,1),size(W,2))...
       && isequal(size(mdes,1),size(B,1),size(A,1),size(A,2),size(xdot_prev,1)))
        error ('input matrix dimensions do not match')
    end
    
%assign to every equation an index    
    u_index = [1:length(u_lim)].';
    I = eye(length(xdot_prev));
    
%compute the remaining moment to compensate
    m = mdes - (I + A*dt)*xdot_prev;
    
%check the type of system and then compute the pseudoinverse 1st step
    order = size(B,2)-size(B,1);

    if order > 0 %over-determined, solution that minimizes the 2norm
        u = inv(W)*B'*inv(B*inv(W)*B')*m;
    elseif order < 0 %under-determined, solution that minimizes the error
        u = inv(B'*B)*B'*m;   
    else %order = 0, sqared thus invertiBrle
        u = inv(B)*m;
    end

%deifne u_sat vector
    u_sat = zeros(length(u),1);
    
    saturated = 0;
%check if the first iteration solution is correct then return    
    if not(any(u <= u_lim(:,1))||any(u >= u_lim(:,2)))  
        return
    end
    
    saturated = 1;
%The software continues only if the solution has to be reduced
%reduce their value
    switch reductionType
        case 1 %truncation
            %takes note of which one are out of their bounds
                u_sat(u < u_lim(:,1)) = 1;
                u_sat(u > u_lim(:,2)) = 1;
                
            %trucate
                u = min(u, u_lim(:,2));
                u = max(u, u_lim(:,1));

        case 2 %scaling solution -> direction preserving
            %reduce
                a = zeros(length(u),1);

                for i = 1:length(u)
                    if u(i)>0
                       a(i) = abs(u(i)/u_lim(i,2));
                    elseif u(i)<0
                       a(i) = abs(u(i)/u_lim(i,1));
                    else
                       a(i) = 0; 
                    end          
                end
                a_max = max(a);
                a_max = max(a_max,1);
                u = u/a_max;
            
            %takes note of which one are out of their bounds
                u_sat(u == u_lim(:,2)) = 1;
                u_sat(u == u_lim(:,1)) = 1;
            
    end
    
return
    
end

== matlab function G_actuatordynamics/error4 ==
  data: e input; error output
function error = error(e)

    error = sum(abs(e));

end

== matlab function G_actuatordynamics/FRAMEWISE CONTROL ALLOCATION simple pseudoinverse3/I ==
  data: u_lim input; u_prev input; udotdt_lim input; I output
function I = computeIntersection(u_lim, u_prev, udotdt_lim)
%check if the matrices are correct
    if not(isequal(size(u_lim,1),size(udotdt_lim,1), size(u_prev,1)))
        error ('input matrix dimensions do not match')
    end

%declare space of intersection
    I = zeros(length(u_lim),2);
    
    I(:,1) = max(-udotdt_lim, u_lim(:,1)-u_prev);
    I(:,2) = min(+udotdt_lim, u_lim(:,2)-u_prev);
    
end

== matlab function G_actuatordynamics/FRAMEWISE CONTROL ALLOCATION simple pseudoinverse3/I1 ==
  data: u_lim input; u input; u output; u_prev input
function u = uCheck(u_lim, u, u_prev)
%check if the matrices are correct
    if not(isequal(size(u_lim,1), size(u,1)))
        error ('input matrix dimensions do not match')
    end

%if computation error occur, correct deflections
    for i = 1:length(u)
        if u(i)+u_prev(i) > u_lim(i,2)
            u(i) = u_lim(i,2)-u_prev(i);
        end
        if u(i)+u_prev(i) < u_lim(i,1)
            u(i) = u_lim(i,1)-u_prev(i);
        end    
    
end

== matlab function G_actuatordynamics/FRAMEWISE CONTROL ALLOCATION simple pseudoinverse3/Pseudoinverse1 ==
  data: mdes input; xdot_prev input; u output; B input; A input; dt input; W input; u_lim input; reductionType input; saturated output
function [u, saturated] = Pseudoinverse(mdes, xdot_prev, B, A, dt, W, u_lim, reductionType)
coder.varsize('u_index', 'Br', 'Wr', 'u_sat');

%check if the matrices are correct
    if not(isequal(size(u_lim,1),size(B,2),size(W,1),size(W,2))...
       && isequal(size(mdes,1),size(B,1),size(A,1),size(A,2),size(xdot_prev,1)))
        error ('input matrix dimensions do not match')
    end
    
%assign to every equation an index    
    u_index = [1:length(u_lim)].';
    I = eye(length(xdot_prev));
    
%compute the remaining moment to compensate
    m = mdes - (I + A*dt)*xdot_prev;
    
%check the type of system and then compute the pseudoinverse 1st step
    order = size(B,2)-size(B,1);

    if order > 0 %over-determined, solution that minimizes the 2norm
        u = inv(W)*B'*inv(B*inv(W)*B')*m;
    elseif order < 0 %under-determined, solution that minimizes the error
        u = inv(B'*B)*B'*m;   
    else %order = 0, sqared thus invertiBrle
        u = inv(B)*m;
    end

%deifne u_sat vector
    u_sat = zeros(length(u),1);
    
    saturated = 0;
%check if the first iteration solution is correct then return    
    if not(any(u <= u_lim(:,1))||any(u >= u_lim(:,2)))  
        return
    end
    
    saturated = 1;
%The software continues only if the solution has to be reduced
%reduce their value
    switch reductionType
        case 1 %truncation
            %takes note of which one are out of their bounds
                u_sat(u < u_lim(:,1)) = 1;
                u_sat(u > u_lim(:,2)) = 1;
                
            %trucate
                u = min(u, u_lim(:,2));
                u = max(u, u_lim(:,1));

        case 2 %scaling solution -> direction preserving
            %reduce
                a = zeros(length(u),1);

                for i = 1:length(u)
                    if u(i)>0
                       a(i) = abs(u(i)/u_lim(i,2));
                    elseif u(i)<0
                       a(i) = abs(u(i)/u_lim(i,1));
                    else
                       a(i) = 0; 
                    end          
                end
                a_max = max(a);
                a_max = max(a_max,1);
                u = u/a_max;
            
            %takes note of which one are out of their bounds
                u_sat(u == u_lim(:,2)) = 1;
                u_sat(u == u_lim(:,1)) = 1;
            
    end
    
return
    
end

== matlab function G_actuatordynamics/error5 ==
  data: e input; error output
function error = error(e)

    error = sum(abs(e));

end

== matlab function G_actuatordynamics/FRAMEWISE CONTROL ALLOCATION simple pseudoinverse4/I ==
  data: u_lim input; u_prev input; udotdt_lim input; I output
function I = computeIntersection(u_lim, u_prev, udotdt_lim)
%check if the matrices are correct
    if not(isequal(size(u_lim,1),size(udotdt_lim,1), size(u_prev,1)))
        error ('input matrix dimensions do not match')
    end

%declare space of intersection
    I = zeros(length(u_lim),2);
    
    I(:,1) = max(-udotdt_lim, u_lim(:,1)-u_prev);
    I(:,2) = min(+udotdt_lim, u_lim(:,2)-u_prev);
    
end

== matlab function G_actuatordynamics/FRAMEWISE CONTROL ALLOCATION simple pseudoinverse4/I1 ==
  data: u_lim input; u input; u output; u_prev input
function u = uCheck(u_lim, u, u_prev)
%check if the matrices are correct
    if not(isequal(size(u_lim,1), size(u,1)))
        error ('input matrix dimensions do not match')
    end

%if computation error occur, correct deflections
    for i = 1:length(u)
        if u(i)+u_prev(i) > u_lim(i,2)
            u(i) = u_lim(i,2)-u_prev(i);
        end
        if u(i)+u_prev(i) < u_lim(i,1)
            u(i) = u_lim(i,1)-u_prev(i);
        end    
    
end
